simulink model "prueba2simpleconmaterialprimerageneracionbuena_1"  (R2017a)
settings: Solver=ode3  StartTime=0.0  StopTime=6.3  FixedStep=5e-3  RelTol=1e-3
values from neighbouring files (symbols this model uses):
  L1 = L1s(L1i)    [beca.m]    (also in calculodepar.m = params.L1)
  L2 = L2s(L2k)    [beca.m]    (also in calculodepar.m = params.L2)
  m = 0.30    (= 0.3)    [calculodepar.m]
  N = m*g - ten*sin(beta)    [calculodepar.m]    (also in main.m = 360)
undefined symbols (not defined in the file or in its folder): corredera, pasador0
libraries: mblibv1 x13
settings Model: Creator=ANGEL  LastModifiedBy=angel
settings DataIOCC: LimitDataPoints=on  SaveFormat=Array  SignalLoggingSaveFormat=ModelDataLogs
settings OptimizationCC: BlockReduction=off  BooleanDataType=off  LifeSpan=inf
settings DebuggingCC: SaveWithParameterizedLinksMsg=none  UnderspecifiedInitializationDetection=Classic  MergeDetectMultiDrivingBlocksExec=none  SignalResolutionControl=TryResolveAllWithWarning  MultiTaskDSMMsg=warning  MultiTaskCondExecSysMsg=none  StateNameClashWarn=warning  SFUnexpectedBacktrackingDiag=warning  SFNoUnconditionalDefaultTransitionDiag=warning  SFExecutionAtInitializationDiag=none
settings HardwareCC: ProdBitPerPointer=32  ProdBitPerSizeT=32  ProdBitPerPtrDiffT=32  ProdLargestAtomicFloat=None  ProdIntDivRoundTo=Undefined  ProdEndianess=Unspecified  ProdWordSize=32  ProdHWDeviceType=32-bit Generic  TargetUnknown=on
settings ModelReferenceCC: PropagateSignalLabelsOutOfModel=off
settings GRTTargetCC: TargetLangStandard=C89/C90 (ANSI)  GeneratePreprocessorConditionals=Disable all
settings ConfigComp: CovMetricSettings=dw  CovHtmlReporting=on  CovSaveCumulativeToWorkspaceVar=on  CovSaveSingleToWorkspaceVar=on  CovExternalEMLEnable=off
settings SimMechanicsCC: VisOnUpdateDiagram=on  VisDuringSimulation=on
settings ConfigurationSet: Description=SimMechanics 2G

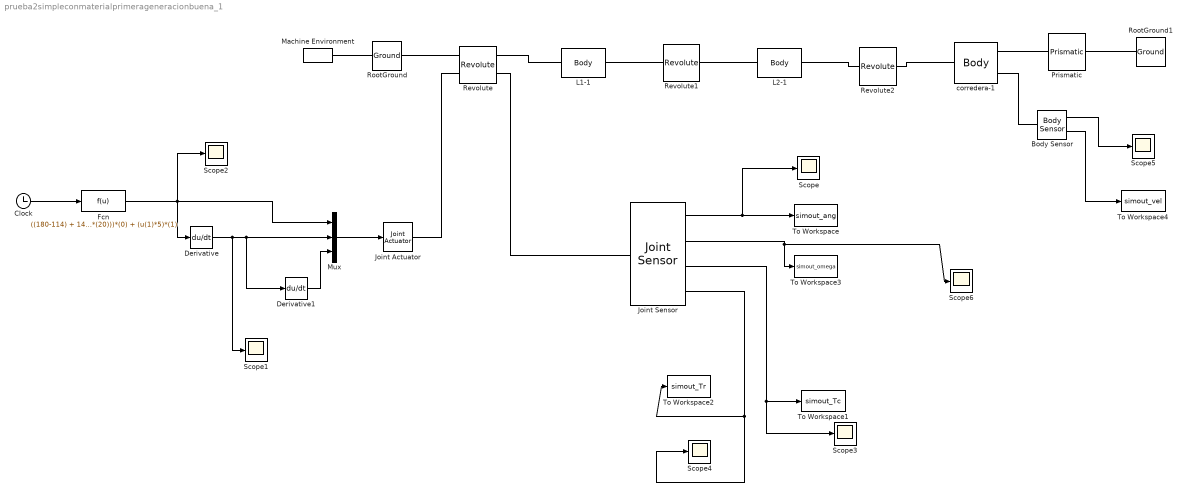
== system prueba2simpleconmaterialprimerageneracionbuena_1 ==
  Body Sensor : mblibv1/Sensors &  Actuators/Body Sensor  UpdateFromCAD=off  PhysicalDomain=Mechanical  PortType=blob  Muxed=off  Pose=off  Angle=on  AngleUnits=deg  ArcVelocity=off  ArcVelocityUnits=deg/s  ArcAcceleration=off  ArcAccelerationUnits=deg/s^2  CoordPosition=off  CoordPositionUnits=m  Velocity=on  VelocityUnits=m/s  Acceleration=on  AccelerationUnits=m/s^2  Quaternion=on  QuaternionDT=off  QuaternionDDT=off  QuaternionUnits=off  OutputVector=[1]  ActiveIO=on  Width=6  DialogClass=MechanicalSensorBlock  ReferenceFrame=Absolute (World)
      settings: SourceProductName=Simscape Multibody  SourceProductBaseCode=MS
  Clock : Clock
  Derivative : Derivative
  Derivative1 : Derivative
  Fcn : Fcn  Expr=((180-114) + 14*sin(2*pi*u(1)*(20)))*(0) + (u(1)*5)*(1)
  Joint Actuator : mblibv1/Sensors &  Actuators/Joint Actuator  UpdateFromCAD=off  PhysicalDomain=Mechanical  PortType=blob  ActuationStyle=Motion  AngleUnits=rad  ArcVelocityUnits=rad/s  ArcAccelerationUnits=rad/s^2  CoordPositionUnits=m  VelocityUnits=m/s  AccelerationUnits=m/s^2  ForceUnits=N  TorqueUnits=N*m  ActiveIO=on  Width=3  DialogClass=MechanicalActuatorBlock  Primitive=R1  ReferenceFrame=Absolute (World)
      settings: SourceProductName=Simscape Multibody  SourceProductBaseCode=MS
  Joint Sensor : mblibv1/Sensors &  Actuators/Joint Sensor  UpdateFromCAD=off  PhysicalDomain=Mechanical  PortType=blob  Muxed=off  Pose=off  Angle=on  AngleUnits=deg  ArcVelocity=on  ArcVelocityUnits=rad/s  ArcAcceleration=off  ArcAccelerationUnits=deg/s^2  CoordPosition=on  CoordPositionUnits=m  Velocity=off  VelocityUnits=m/s  Acceleration=off  AccelerationUnits=m/s^2  Quaternion=on  QuaternionDT=off  QuaternionDDT=off  QuaternionUnits=off  OutputVector=[1]  ActiveIO=on  Width=6  DialogClass=MechanicalSensorBlock  Primitive=R1  Force=off  ForceUnits=N  Torque=on  TorqueUnits=N*m  ReferenceFrame=Absolute (World)  ReactionSensedSide=Base  ReactionReferenceFrame=Absolute (World)  ReactionForce=off  ReactionForceUnits=N  ReactionMoment=on  ReactionMomentUnits=N*m
      settings: SourceProductName=Simscape Multibody  SourceProductBaseCode=MS
  L1-1 : mblibv1/Bodies/Body  LConnTagsString=CS2  RConnTagsString=CS3  UpdateFromCAD=on  PMImportedID=L1-1  DialogClass=MechanicalBodyBlock  Mass=0.00593014  MassUnits=kg  InertiaUnits=kg*m^2  Inertia=[1.04021e-06,0,0;0,1.07865e-06,0;0,0,6.31529e-08]  Shape=Cylinder  ShapeDims=[1 1]  ShapeUnits=m  ShapeUse=false  Density=1  DensityUnits=kg/m^3  DensityUse=false  GraphicsMode=CONVHULL  GraphicsFileName=prueba2simpleconmaterialprimerageneracionbuena - L1-1.STL  BodyColorSelMode=COLORPALETTE  BodyColor=[0 0 0]  AttachedToCS=CG  CG=Right$CG$[0.02 0 0]$WORLD$WORLD$m$[0.990758 0 0.135645;0 1 0;-0.135645 0 0.990758]$3x3 Transform$rad$WORLD$false$L1-1::CG(AUTOGEN)  WorkingFrames=Left$CS2$[0 0 0]$WORLD$WORLD$m$[0 0 0]$Euler X-Y-Z$rad$WORLD$true$L1-1:-:pasador0.5-1::L1-1(AUTOGEN)#Right$CS3$[0.04 0 0]$WORLD$WORLD$m$[0 0 0]$Euler X-Y-Z$rad$WORLD$true$L1-1:-:L2-1::L1-1(AUTOGEN)  CGPos=[0.02 0 0]  CGRot=[0.990758 0 0.135645;0 1 0;-0.135645 0 0.990758]  CS0Pos=[]  CS0Rot=[]  CS1Pos=[]  CS1Rot=[]  CS2Pos=[0 0 0]  CS2Rot=[0 0 0]  CS3Pos=[0.04 0 0]  CS3Rot=[0 0 0]  CS4Pos=[]  CS4Rot=[]  CS5Pos=[]  CS5Rot=[]  CS6Pos=[]  CS6Rot=[]  CS7Pos=[]  CS7Rot=[]  CS8Pos=[]  CS8Rot=[]  CS9Pos=[]  CS9Rot=[]  CS10Pos=[]  CS10Rot=[]  CS11Pos=[]  CS11Rot=[]  CS12Pos=[]  CS12Rot=[]  CS13Pos=[]  CS13Rot=[]  CS14Pos=[]  CS14Rot=[]  CS15Pos=[]  CS15Rot=[]  CS16Pos=[]  CS16Rot=[]  CS17Pos=[]  CS17Rot=[]  CS18Pos=[]  CS18Rot=[]  CS19Pos=[]  CS19Rot=[]  CS20Pos=[]  CS20Rot=[]
      settings: SourceProductName=Simscape Multibody  SourceProductBaseCode=MS
  L2-1 : mblibv1/Bodies/Body  LConnTagsString=CS2  RConnTagsString=CS3  UpdateFromCAD=on  PMImportedID=L2-1  DialogClass=MechanicalBodyBlock  Mass=0.00998014  MassUnits=kg  InertiaUnits=kg*m^2  Inertia=[4.69227e-06,0,0;0,4.75602e-06,0;0,0,1.0534e-07]  Shape=Cylinder  ShapeDims=[1 1]  ShapeUnits=m  ShapeUse=false  Density=1  DensityUnits=kg/m^3  DensityUse=false  GraphicsMode=CONVHULL  GraphicsFileName=prueba2simpleconmaterialprimerageneracionbuena - L2-1.STL  BodyColorSelMode=COLORPALETTE  BodyColor=[0 0 0]  AttachedToCS=CG  CG=Right$CG$[0.035 0 0]$World$CS2$m$[0.996991 0 -0.0775113;0 1 0;0.0775113 0 0.996991]$3x3 Transform$rad$WORLD$false$L2-1::CG(AUTOGEN)  WorkingFrames=Left$CS2$[0 0 0]$World$Adjoining$m$[1 0 0;0 1 0;0 0 1]$3x3 Transform$rad$WORLD$true$L1-1:-:L2-1::L2-1(AUTOGEN)#Right$CS3$[0.07 0 0]$CS2$CS2$m$[1 0 0;0 1 0;0 0 1]$3x3 Transform$rad$WORLD$true$L2-1:-:corredera-1::L2-1(AUTOGEN)  CGPos=[0.035 0 0]  CGRot=[0.996991 0 -0.0775113;0 1 0;0.0775113 0 0.996991]  CS0Pos=[]  CS0Rot=[]  CS1Pos=[]  CS1Rot=[]  CS2Pos=[0 0 0]  CS2Rot=[1 0 0;0 1 0;0 0 1]  CS3Pos=[0.07 0 0]  CS3Rot=[1 0 0;0 1 0;0 0 1]  CS4Pos=[]  CS4Rot=[]  CS5Pos=[]  CS5Rot=[]  CS6Pos=[]  CS6Rot=[]  CS7Pos=[]  CS7Rot=[]  CS8Pos=[]  CS8Rot=[]  CS9Pos=[]  CS9Rot=[]  CS10Pos=[]  CS10Rot=[]  CS11Pos=[]  CS11Rot=[]  CS12Pos=[]  CS12Rot=[]  CS13Pos=[]  CS13Rot=[]  CS14Pos=[]  CS14Rot=[]  CS15Pos=[]  CS15Rot=[]  CS16Pos=[]  CS16Rot=[]  CS17Pos=[]  CS17Rot=[]  CS18Pos=[]  CS18Rot=[]  CS19Pos=[]  CS19Rot=[]  CS20Pos=[]  CS20Rot=[]
      settings: SourceProductName=Simscape Multibody  SourceProductBaseCode=MS
  Machine Environment : mblibv1/Bodies/Machine Environment  PortType=env  PhysicalDomain=Mechanical  DialogTemplateClass=MECH.MachineEnvironment  SyncWhenCopied=off  Gravity=[0 0 0]  GravityUnits=m/s^2  GravityAsSignal=off  Dimensionality=Auto-detect  AnalysisType=Forward dynamics  LinearAssemblyTolerance=1e-3  LinearAssemblyToleranceUnits=m  AngularAssemblyTolerance=1e-3  AngularAssemblyToleranceUnits=rad  ConstraintSolverType=Tolerancing  ConstraintRelTolerance=1e-4  ConstraintAbsTolerance=1e-4  UseRobustSingularityHandling=off  RedundancyAnalysisToleranceType=Automatically select tolerance  RedundancyAnalysisTolerance=1e-14  StatePerturbationType=Fixed  PerturbationSize=1e-5  VisualizeMachine=on  BodyVisualizationType=Use model default body geometries  BodyColorSelMode=Use model default  DefaultBodyColor=[1 0 0]
      settings: SourceProductName=Simscape Multibody  SourceProductBaseCode=MS
  Mux : Mux  Inputs=3
  Prismatic : mblibv1/Joints/Prismatic  LConnTagsString=__newl0  RConnTagsString=__newr0  UpdateFromCAD=off  NumSAPorts=0  CutJoint=off  MarkAsCut=off  Primitives=prismatic  PrimitiveProps=P1$World$[1 0 0]$prismatic  DialogClass=JointBlock  P1Axis=[1 0 0]
      settings: SourceProductName=Simscape Multibody  SourceProductBaseCode=MS
  Revolute : mblibv1/Joints/Revolute  LConnTagsString=__newl0|SA1  RConnTagsString=__newr0|SA1  UpdateFromCAD=on  PMImportedID=L1-1:-:pasador0.5-1  NumSAPorts=2  CutJoint=off  MarkAsCut=off  Primitives=prismatic  PrimitiveProps=R1$World$[0,0,1]$revolute  DialogClass=JointBlock  R1Axis=[0,0,1]
      settings: SourceProductName=Simscape Multibody  SourceProductBaseCode=MS
  Revolute1 : mblibv1/Joints/Revolute  LConnTagsString=__newl0  RConnTagsString=__newr0  UpdateFromCAD=on  PMImportedID=L1-1:-:L2-1  NumSAPorts=0  CutJoint=off  MarkAsCut=off  Primitives=prismatic  PrimitiveProps=R1$World$[0,0,1]$revolute  DialogClass=JointBlock  R1Axis=[0,0,1]
      settings: SourceProductName=Simscape Multibody  SourceProductBaseCode=MS
  Revolute2 : mblibv1/Joints/Revolute  LConnTagsString=__newl0  RConnTagsString=__newr0  UpdateFromCAD=on  PMImportedID=L2-1:-:corredera-1  NumSAPorts=0  CutJoint=off  MarkAsCut=off  Primitives=prismatic  PrimitiveProps=R1$World$[0,0,1]$revolute  DialogClass=JointBlock  R1Axis=[0,0,1]
      settings: SourceProductName=Simscape Multibody  SourceProductBaseCode=MS
  RootGround : mblibv1/Bodies/Ground  UpdateFromCAD=on  PMImportedID=RootGround  LeftPortType=env  RightPortType=workingframe  PhysicalDomain=Mechanical  DialogClass=GroundBlock  CoordPosition=[0 0 0]  CoordPositionUnits=m  StateVectorMgrId=0  MachineId=[1 0]  ShowEnvPort=on  ParameterChecksum=[3452590705, 1352005729, 1677675091, 1007898850]  TopologyChecksum=[1527311189, 4239167037, 1660867997, 272355560]
      settings: SourceProductName=Simscape Multibody  SourceProductBaseCode=MS
  RootGround1 : mblibv1/Bodies/Ground  UpdateFromCAD=on  LeftPortType=env  RightPortType=workingframe  PhysicalDomain=Mechanical  DialogClass=GroundBlock  CoordPosition=[0.11 0 0]  CoordPositionUnits=m  StateVectorMgrId=-1  MachineId=[0 0]  ShowEnvPort=off  ParameterChecksum=[0 0 0 0]  TopologyChecksum=[0 0 0 0]
      settings: SourceProductName=Simscape Multibody  SourceProductBaseCode=MS
  Scope{,1..6} (7 alike) : Scope
  To Workspace : ToWorkspace  VariableName=simout_ang  SaveFormat=Timeseries  SampleTime=-1
  To Workspace1 : ToWorkspace  VariableName=simout_Tc  SaveFormat=Timeseries  SampleTime=-1
  To Workspace2 : ToWorkspace  VariableName=simout_Tr  SaveFormat=Timeseries  SampleTime=-1
  To Workspace3 : ToWorkspace  VariableName=simout_omega  SaveFormat=Timeseries  SampleTime=-1
  To Workspace4 : ToWorkspace  VariableName=simout_vel  SaveFormat=Timeseries  SampleTime=-1
  corredera-1 : mblibv1/Bodies/Body  LConnTagsString=CS3  RConnTagsString=CS1|CS2  UpdateFromCAD=on  PMImportedID=corredera-1  DialogClass=MechanicalBodyBlock  Mass=3  MassUnits=kg  InertiaUnits=kg*m^2  Inertia=[5.21811e-07,0,0;0,3.55655e-07,0;0,0,6.05651e-07]*0  Shape=Cylinder  ShapeDims=[1 1]  ShapeUnits=m  ShapeUse=false  Density=1  DensityUnits=kg/m^3  DensityUse=false  GraphicsMode=CONVHULL  GraphicsFileName=prueba2simpleconmaterialprimerageneracionbuena - corredera-1.STL  BodyColorSelMode=COLORPALETTE  BodyColor=[1 0 0]  AttachedToCS=CG  CG=Right$CG$[0.15 0 0]$World$CS3$m$[-1 0 0;0 1 0;0 0 -1]$3x3 Transform$rad$WORLD$false$corredera-1::CG(AUTOGEN)  WorkingFrames=Left$CS3$[0 0 0]$World$Adjoining$m$[1 0 0;0 1 0;0 0 1]$3x3 Transform$rad$WORLD$true$L2-1:-:corredera-1::corredera-1(AUTOGEN)#Right$CS1$[0 0 0]$World$CS3$m$[1 0 0;0 1 0;0 0 1]$3x3 Transform$rad$WORLD$true$none#Right$CS2$[0.3 0 0]$World$CS3$m$[-1 0 0;0 1 0;0 0 -1]$3x3 Transform$rad$WORLD$true$none  CGPos=[0.15 0 0]  CGRot=[-1 0 0;0 1 0;0 0 -1]  CS0Pos=[]  CS0Rot=[]  CS1Pos=[0 0 0]  CS1Rot=[1 0 0;0 1 0;0 0 1]  CS2Pos=[0.3 0 0]  CS2Rot=[-1 0 0;0 1 0;0 0 -1]  CS3Pos=[0 0 0]  CS3Rot=[1 0 0;0 1 0;0 0 1]  CS4Pos=[]  CS4Rot=[]  CS5Pos=[]  CS5Rot=[]  CS6Pos=[]  CS6Rot=[]  CS7Pos=[]  CS7Rot=[]  CS8Pos=[]  CS8Rot=[]  CS9Pos=[]  CS9Rot=[]  CS10Pos=[]  CS10Rot=[]  CS11Pos=[]  CS11Rot=[]  CS12Pos=[]  CS12Rot=[]  CS13Pos=[]  CS13Rot=[]  CS14Pos=[]  CS14Rot=[]  CS15Pos=[]  CS15Rot=[]  CS16Pos=[]  CS16Rot=[]  CS17Pos=[]  CS17Rot=[]  CS18Pos=[]  CS18Rot=[]  CS19Pos=[]  CS19Rot=[]  CS20Pos=[]  CS20Rot=[]
      settings: SourceProductName=Simscape Multibody  SourceProductBaseCode=MS
  wires:
  Mux/1 -> Joint Actuator/1
  Derivative1/1 -> Mux/3
  Joint Sensor/1 -> Scope/1, To Workspace/1
  Clock/1 -> Fcn/1
  Fcn/1 -> Derivative/1, Mux/1, Scope2/1
  Derivative/1 -> Scope1/1, Derivative1/1, Mux/2
  Body Sensor/1 -> Scope5/1
  Joint Sensor/3 -> Scope3/1, To Workspace1/1
  Joint Sensor/4 -> Scope4/1, To Workspace2/1
  Joint Sensor/2 -> Scope6/1, To Workspace3/1
  Body Sensor/2 -> To Workspace4/1
  connections:
  RootGround/RConn1 -- Revolute/LConn1
  Revolute1/RConn1 -- L2-1/LConn1
  L2-1/RConn1 -- Revolute2/LConn1
  RootGround/LConn1 -- Machine Environment/RConn1
  Prismatic/RConn1 -- RootGround1/RConn1
  Revolute/RConn1 -- L1-1/LConn1
  L1-1/RConn1 -- Revolute1/LConn1
  Revolute2/RConn1 -- corredera-1/LConn1
  corredera-1/RConn1 -- Prismatic/LConn1
  Joint Sensor/LConn1 -- Revolute/RConn2
  Joint Actuator/RConn1 -- Revolute/LConn2
  Body Sensor/LConn1 -- corredera-1/RConn2
